simulink model "trabalhofinal_vR2016a"  (R2016a)
settings: Solver=FixedStepDiscrete  StartTime=0.0  StopTime=0.5  FixedStep=0.1e-6  MaxStep=50e-6
undefined symbols (not defined in the file): DiscIntNeverNeededParam, Ipac0, Vpac0
libraries: powerlib x36, simulink x19, fuzblock x7, powerlib_extras x2, powerlib_meascontrol x2
(part 3 of 3)

== system trabalhofinal_vR2016a/PV array Fuzzy/DSOGI1/Calcula Impedância2/DSOGI (Tensão)/SOGI BPF(alfa)  ==
  wr : Inport
  fal : Inport  Port=2
  Gain : Gain  Gain=1/2
  Gain2 : Gain  Gain=k
  Integrator : Integrator  InitialCondition=int1_v
  Integrator1 : Integrator  InitialCondition=int2_v
  Product : Product
  Product1 : Product
  Sum : Sum  Inputs=-+|
  Sum2 : Sum  Inputs=|+-
  fal' : Outport
  qfal' : Outport  Port=2
  wires:
  Integrator1/1 -> qfal'/1, Sum2/2
  wr/1 -> Product1/1, Product/1
  Sum2/1 -> Product/2
  Sum/1 -> Gain2/1
  Product1/1 -> Integrator1/1
  Integrator/1 -> fal'/1, Sum/1, Product1/2
  Gain2/1 -> Sum2/1
  Product/1 -> Integrator/1
  Gain/1 -> Sum/2
  fal/1 -> Gain/1

== system trabalhofinal_vR2016a/PV array Fuzzy/DSOGI1/Calcula Impedância2/PLL/abc2dq0 PSIM ==
  Falbe : Inport
  wt : Inport  Port=2
  Fcn1 : Fcn  Expr=u(1)*cos(u(3))+u(2)*sin(u(3))
  Fcn2 : Fcn  Expr=u(1)*sin(u(3))-u(2)*cos(u(3))
  Mux : Mux  Inputs=2
  Fq : Outport
  Fd : Outport  Port=2
  wires:
  Mux/1 -> Fcn1/1, Fcn2/1
  wt/1 -> Mux/2
  Fcn2/1 -> Fd/1
  Fcn1/1 -> Fq/1
  Falbe/1 -> Mux/1

== system trabalhofinal_vR2016a/PV array PI/DSOGI1/Calcula Impedância2/DSOGI (Corrente)/SOGI BPF (beta) ==
  wr : Inport
  fbe : Inport  Port=2
  Gain : Gain  Gain=1/2
  Gain2 : Gain  Gain=k
  Integrator : Integrator  InitialCondition=int3_i
  Integrator1 : Integrator  InitialCondition=int4_i
  Product : Product
  Product1 : Product
  Sum : Sum  Inputs=-+|
  Sum2 : Sum  Inputs=|+-
  fbe' : Outport
  qfbe' : Outport  Port=2
  wires:
  fbe/1 -> Gain/1
  Gain/1 -> Sum/2
  Product/1 -> Integrator/1
  Gain2/1 -> Sum2/1
  Integrator/1 -> Product1/2, Sum/1, fbe'/1
  Product1/1 -> Integrator1/1
  Sum/1 -> Gain2/1
  Sum2/1 -> Product/2
  wr/1 -> Product/1, Product1/1
  Integrator1/1 -> Sum2/2, qfbe'/1

== system trabalhofinal_vR2016a/PV array PI/DSOGI1/Calcula Impedância2/DSOGI (Corrente)/SOGI BPF(alfa)  ==
  wr : Inport
  fal : Inport  Port=2
  Gain : Gain  Gain=1/2
  Gain2 : Gain  Gain=k
  Integrator : Integrator  InitialCondition=int1_i
  Integrator1 : Integrator  InitialCondition=int2_i
  Product : Product
  Product1 : Product
  Sum : Sum  Inputs=-+|
  Sum2 : Sum  Inputs=|+-
  fal' : Outport
  qfal' : Outport  Port=2
  wires:
  Integrator1/1 -> qfal'/1, Sum2/2
  wr/1 -> Product1/1, Product/1
  Sum2/1 -> Product/2
  Sum/1 -> Gain2/1
  Product1/1 -> Integrator1/1
  Integrator/1 -> fal'/1, Sum/1, Product1/2
  Gain2/1 -> Sum2/1
  Product/1 -> Integrator/1
  Gain/1 -> Sum/2
  fal/1 -> Gain/1

== system trabalhofinal_vR2016a/PV array PI/DSOGI1/Calcula Impedância2/DSOGI (Tensão)/SOGI BPF (beta) ==
  wr : Inport
  fbe : Inport  Port=2
  Gain : Gain  Gain=1/2
  Gain2 : Gain  Gain=k
  Integrator : Integrator  InitialCondition=int3_v
  Integrator1 : Integrator  InitialCondition=int4_v
  Product : Product
  Product1 : Product
  Sum : Sum  Inputs=-+|
  Sum2 : Sum  Inputs=|+-
  fbe' : Outport
  qfbe' : Outport  Port=2
  wires:
  fbe/1 -> Gain/1
  Gain/1 -> Sum/2
  Product/1 -> Integrator/1
  Gain2/1 -> Sum2/1
  Integrator/1 -> Product1/2, Sum/1, fbe'/1
  Product1/1 -> Integrator1/1
  Sum/1 -> Gain2/1
  Sum2/1 -> Product/2
  wr/1 -> Product/1, Product1/1
  Integrator1/1 -> Sum2/2, qfbe'/1

== system trabalhofinal_vR2016a/PV array PI/DSOGI1/Calcula Impedância2/DSOGI (Tensão)/SOGI BPF(alfa)  ==
  wr : Inport
  fal : Inport  Port=2
  Gain : Gain  Gain=1/2
  Gain2 : Gain  Gain=k
  Integrator : Integrator  InitialCondition=int1_v
  Integrator1 : Integrator  InitialCondition=int2_v
  Product : Product
  Product1 : Product
  Sum : Sum  Inputs=-+|
  Sum2 : Sum  Inputs=|+-
  fal' : Outport
  qfal' : Outport  Port=2
  wires:
  Integrator1/1 -> qfal'/1, Sum2/2
  wr/1 -> Product1/1, Product/1
  Sum2/1 -> Product/2
  Sum/1 -> Gain2/1
  Product1/1 -> Integrator1/1
  Integrator/1 -> fal'/1, Sum/1, Product1/2
  Gain2/1 -> Sum2/1
  Product/1 -> Integrator/1
  Gain/1 -> Sum/2
  fal/1 -> Gain/1

== system trabalhofinal_vR2016a/PV array PI/DSOGI1/Calcula Impedância2/PLL/abc2dq0 PSIM ==
  Falbe : Inport
  wt : Inport  Port=2
  Fcn1 : Fcn  Expr=u(1)*cos(u(3))+u(2)*sin(u(3))
  Fcn2 : Fcn  Expr=u(1)*sin(u(3))-u(2)*cos(u(3))
  Mux : Mux  Inputs=2
  Fq : Outport
  Fd : Outport  Port=2
  wires:
  Mux/1 -> Fcn1/1, Fcn2/1
  wt/1 -> Mux/2
  Fcn2/1 -> Fd/1
  Fcn1/1 -> Fq/1
  Falbe/1 -> Mux/1
